simulink model "fzpi1"  (R2022b)
settings: Solver=VariableStepAuto  StartTime=0.0  StopTime=1.0  RelTol=1e-3
values from neighbouring files (symbols this model uses):
  K1 = kp / (a * Ke)    (= 20)    [main.m]
  Kd = a*Ke    (= 0.0666666666667)    [main.m]
  wmax = 150    [main.m]
libraries: fuzblock x1
settings Model: Creator=karam  LastModifiedBy=kmpouzio
settings SolverCC: AlgebraicLoopSolver=TrustRegion
settings DebuggingCC: UnconnectedInputMsg=warning  UnconnectedOutputMsg=warning  UnconnectedLineMsg=warning  SFMachineParentedDataDiag=warning
settings ModelReferenceCC: EnableRefExpFcnMdlSchedulingChecks=on

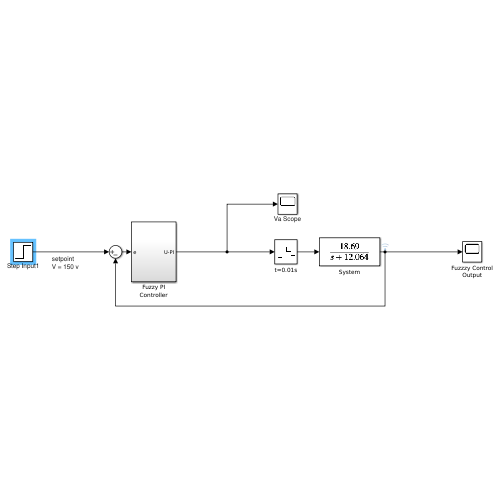
[thumbnail: Simulink's stored preview of the top-level diagram]
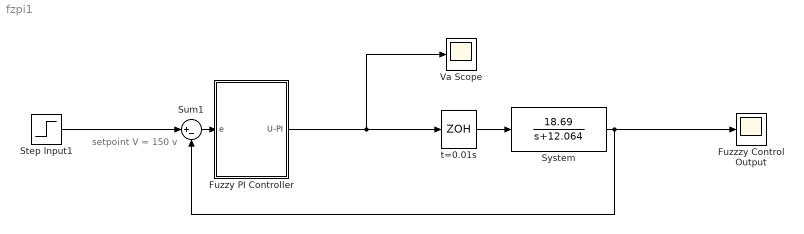
== system fzpi1 ==
  note: setpoint
      | V = 150 v
  Fuzzy PI Controller : Subsystem
  Fuzzzy Control Output : Scope
  Step Input1 : Step  Time=0  After=wmax  SampleTime=0.1
  Sum1 : Sum  Inputs=|+-
  System : TransferFcn  Numerator=[18.69]  Denominator=[1 12.064]
  Va Scope : Scope
  t=0.01s : ZeroOrderHold  SampleTime=0.01
  wires:
  Sum1/1 -> Fuzzy PI Controller/1(e)
  System/1 -> Sum1/2, Fuzzzy Control Output/1
  Step Input1/1 -> Sum1/1
  t=0.01s/1 -> System/1
  Fuzzy PI Controller/1(U-PI) -> Va Scope/1, t=0.01s/1

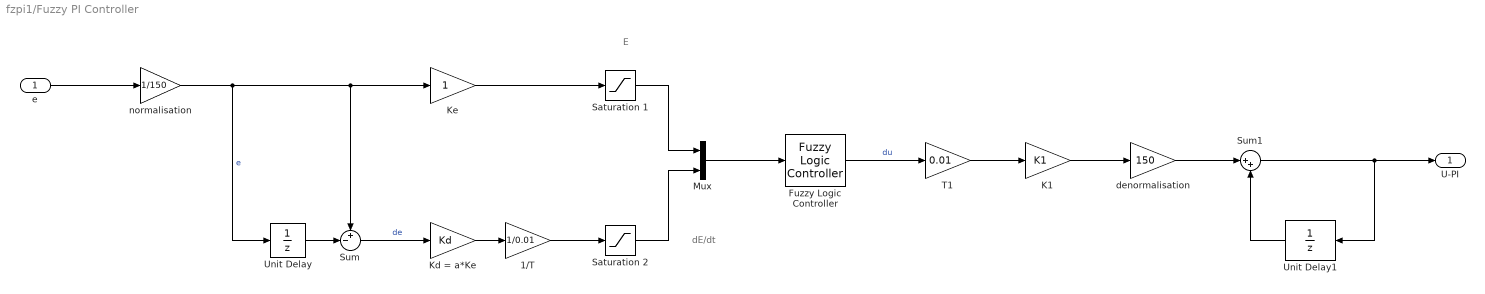
== system fzpi1/Fuzzy PI Controller ==
  note: dE/dt
  note: E
  e : Inport
  1/T : Gain  Gain=1/0.01
  Fuzzy Logic Controller : fuzblock/Fuzzy Logic  Controller  FIS='FLC07.fis'  OutputSampleNumber=101  DataType=double  FuzzifiedInputs=off  RuleFiringStrengths=off  RuleOutputs=off  AggregatedOutputs=off  SimulateUsing=Interpreted execution  OutOfRangeInputValueMessage=warning  NoRuleFiredMessage=warning  EmptyOutputFuzzySetMessage=warning
  K1 : Gain  Gain=K1
  Kd = a*Ke : Gain  Gain=Kd
  Ke : Gain
  Mux : Mux  Inputs=2
  Saturation 1 : Saturate  UpperLimit=1  LowerLimit=-1
  Saturation 2 : Saturate  UpperLimit=1  LowerLimit=-1
  Sum : Sum  Inputs=+-|
  Sum1 : Sum  Inputs=|++
  T1 : Gain  Gain=0.01
  Unit Delay : UnitDelay  SampleTime=0.01  HasFrameUpgradeWarning=on
  Unit Delay1 : UnitDelay  SampleTime=-1  HasFrameUpgradeWarning=on
  denormalisation : Gain  Gain=150
  normalisation : Gain  Gain=1/150
  U-PI : Outport  VectorParamsAs1DForOutWhenUnconnected=off
  wires:
  denormalisation/1 -> Sum1/1
  K1/1 -> denormalisation/1
  e/1 -> normalisation/1
  T1/1 -> K1/1
  Sum1/1 -> Unit Delay1/1, U-PI/1
  Unit Delay1/1 -> Sum1/2
  Ke/1 -> Saturation 1/1
  Kd = a*Ke/1 -> 1/T/1
  normalisation/1 -> Ke/1, Sum/1, Unit Delay/1  "e"
  Sum/1 -> Kd = a*Ke/1  "de"
  Fuzzy Logic Controller/1 -> T1/1  "du"
  Unit Delay/1 -> Sum/2
  Saturation 2/1 -> Mux/2
  Saturation 1/1 -> Mux/1
  1/T/1 -> Saturation 2/1
  Mux/1 -> Fuzzy Logic Controller/1
